simulink model "Sistem1"  (R2015b)
settings: Solver=ode45  StartTime=0.0  StopTime=10.0  RelTol=1e-3
undefined symbols (not defined in the file or in its folder): b, k, m
settings Model: Creator=ETF1-13  LastModifiedBy=user
settings DataIOCC: SaveFormat=Array
settings HardwareCC: ProdBitPerPointer=32  ProdLargestAtomicFloat=None  ProdIntDivRoundTo=Undefined  ProdEndianess=Unspecified  ProdWordSize=32  ProdHWDeviceType=32-bit Generic
settings GRTTargetCC: GeneratePreprocessorConditionals=Disable all
settings ConfigComp: CovModelRefEnable=Off

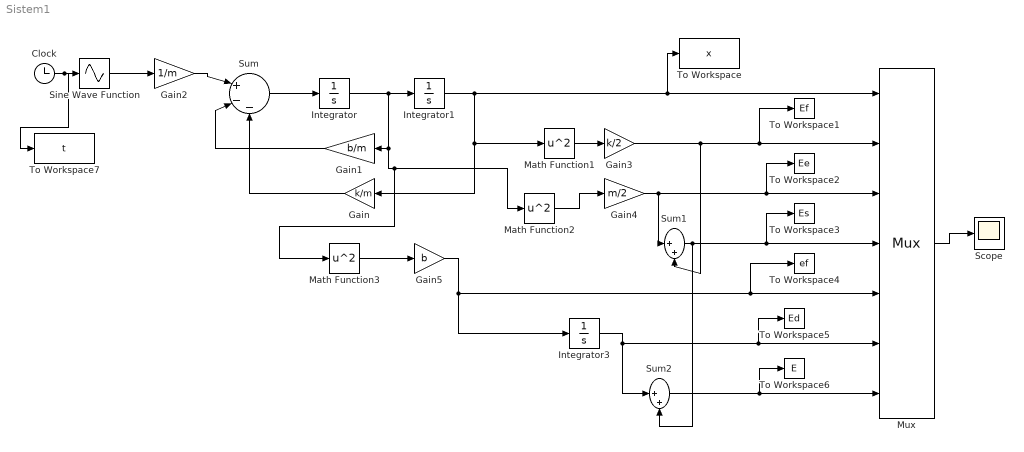
== system Sistem1 ==
  Clock : Clock
  Gain : Gain  Gain=k/m
  Gain1 : Gain  Gain=b/m
  Gain2 : Gain  Gain=1/m
  Gain3 : Gain  Gain=k/2
  Gain4 : Gain  Gain=m/2
  Gain5 : Gain  Gain=b
  Integrator : Integrator  InitialCondition=1
  Integrator1 : Integrator  InitialCondition=1
  Integrator3 : Integrator
  Math Function1 : Math  Operator=square  SaturateOnIntegerOverflow=on
  Math Function2 : Math  Operator=square  SaturateOnIntegerOverflow=on
  Math Function3 : Math  Operator=square  SaturateOnIntegerOverflow=on
  Mux : Mux  Inputs=7
  Scope : Scope
  Sine Wave Function : Sin  TimeSource=Use external signal  Frequency=6.28  SampleTime=0
  Sum : Sum  Inputs=|+--
  Sum1 : Sum  Inputs=|++
  Sum2 : Sum  Inputs=|++
  To Workspace : ToWorkspace  VariableName=x  SampleTime=-1
  To Workspace1 : ToWorkspace  VariableName=Ef  SampleTime=-1
  To Workspace2 : ToWorkspace  VariableName=Ee  SampleTime=-1
  To Workspace3 : ToWorkspace  VariableName=Es  SampleTime=-1
  To Workspace4 : ToWorkspace  VariableName=ef  SampleTime=-1
  To Workspace5 : ToWorkspace  VariableName=Ed  SampleTime=-1
  To Workspace6 : ToWorkspace  VariableName=E  SampleTime=-1
  To Workspace7 : ToWorkspace  VariableName=t  SampleTime=-1
  wires:
  Sum/1 -> Integrator/1
  Integrator1/1 -> Math Function1/1, Gain/1, Mux/1, To Workspace/1
  Gain/1 -> Sum/3
  Gain1/1 -> Sum/2
  Sine Wave Function/1 -> Gain2/1
  Gain2/1 -> Sum/1
  Clock/1 -> To Workspace7/1, Sine Wave Function/1
  Math Function1/1 -> Gain3/1
  Gain3/1 -> Sum1/2, Mux/2, To Workspace1/1
  Integrator/1 -> Math Function3/1, Math Function2/1, Gain1/1, Integrator1/1
  Math Function2/1 -> Gain4/1
  Gain4/1 -> Sum1/1, Mux/3, To Workspace2/1
  Sum1/1 -> Mux/4, To Workspace3/1, Sum2/2
  Integrator3/1 -> Sum2/1, Mux/6, To Workspace5/1
  Sum2/1 -> Mux/7, To Workspace6/1
  Mux/1 -> Scope/1
  Gain5/1 -> Integrator3/1, Mux/5, To Workspace4/1
  Math Function3/1 -> Gain5/1
